simulink model "pendulum2d"  (R2017a)
settings: Solver=FixedStepAuto  StartTime=0.0  StopTime=10.0  FixedStep=1e-3  RelTol=1e-3
values from neighbouring files (symbols this model uses):
  theta_init = 15 *pi/180    (= 0.261799387799)    [initialize_2Dnonlinear_system.m]
libraries: sldrtlib x1
settings Model: Creator=Jan  LastModifiedBy=Jan

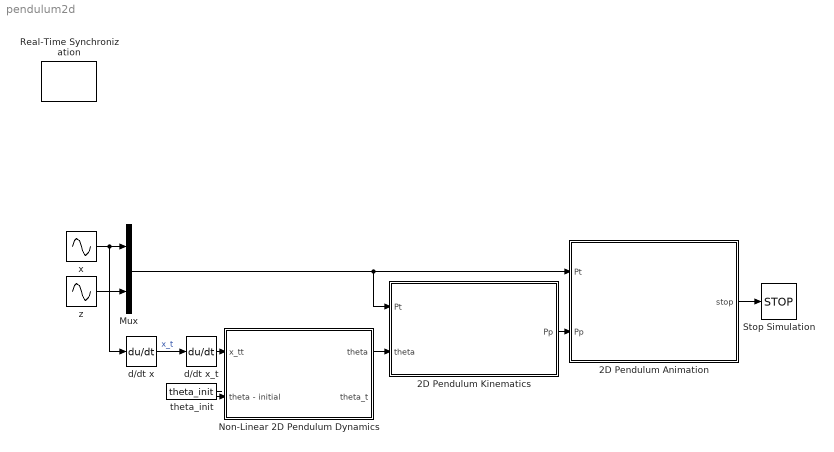
== system pendulum2d ==
  2D Pendulum Animation : MATLAB Function  TreatAsAtomicUnit=on  SystemSampleTime=0.05
  2D Pendulum Kinematics : MATLAB Function  TreatAsAtomicUnit=on
  Mux : Mux  Inputs=2
  Non-Linear 2D Pendulum Dynamics : Subsystem
  Real-Time Synchronization : sldrtlib/Real-Time Synchronization  SampleTime=0.05  MaxMissedTicks=10  ShowMissedTicks=off  YieldWhenWaiting=off
  Stop Simulation : Stop
  d/dt x : Derivative
  d/dt x_t : Derivative
  theta_init : Constant  Value=theta_init
  x : Sin  Frequency=2*pi*0.1  SampleTime=0
  z : Sin  Frequency=2*pi*0.1  SampleTime=0
  wires:
  theta_init/1 -> Non-Linear 2D Pendulum Dynamics/2(theta - initial)
  d/dt x_t/1 -> Non-Linear 2D Pendulum Dynamics/1(x_tt)
  d/dt x/1 -> d/dt x_t/1  "x_t"
  2D Pendulum Animation/1(stop) -> Stop Simulation/1
  x/1 -> d/dt x/1, Mux/1
  z/1 -> Mux/2
  Non-Linear 2D Pendulum Dynamics/1(theta) -> 2D Pendulum Kinematics/2(theta)
  Mux/1 -> 2D Pendulum Animation/1(Pt), 2D Pendulum Kinematics/1(Pt)
  2D Pendulum Kinematics/1(Pp) -> 2D Pendulum Animation/2(Pp)

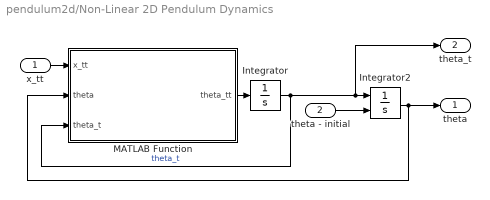
== system pendulum2d/Non-Linear 2D Pendulum Dynamics ==
  x_tt : Inport
  theta - initial : Inport  Port=2
  Integrator : Integrator
  Integrator2 : Integrator  InitialConditionSource=external
  MATLAB Function : MATLAB Function  TreatAsAtomicUnit=on
  theta : Outport
  theta_t : Outport  Port=2
  wires:
  Integrator2/1 -> theta/1, MATLAB Function/2(theta)
  theta - initial/1 -> Integrator2/2
  MATLAB Function/1(theta_tt) -> Integrator/1
  x_tt/1 -> MATLAB Function/1(x_tt)
  Integrator/1 -> theta_t/1, Integrator2/1, MATLAB Function/3(theta_t)  "theta_t"

== matlab function pendulum2d/Non-Linear 2D Pendulum Dynamics/MATLAB Function ==
  data: x_tt input; theta input; theta_tt output; theta_t input
function theta_tt = pendulum2D_dynamics(x_tt, theta, theta_t)
    
    % Constants
    g = 9.81;   % Gravity
    L = 2.0;    % Wire length
    
    % Pendulum ODE
    theta_tt = (-g*sin(theta) - cos(theta)*x_tt)/L;

== matlab function pendulum2d/2D Pendulum Kinematics ==
  data: Pt input; theta input; Pp output
function Pp = pendulum_kinematics(Pt, theta)
    
    % Constants
    g = 9.81;   % Gravity
    L = 2.0;    % Wire length
    
    % Pendulum Kinematics
    Pp = Pt + L*[sin(theta); -cos(theta)];

== matlab function pendulum2d/2D Pendulum Animation ==
  data: Pt input; stop output; Pp input
function stop = SimulinkPendulumPlot(Pt, Pp)
    % Creates a 2D-animation for the pendulum motion
    % Input:
    %   xt :   Position of tool-point
    %   theta : Euler angle of pendulum
    % Output:
    %   stop : Bool value to stop the animation
    
    % Persistent variables, to only be initialized once
    persistent h;           % Plot
    persistent L;
    
    stop = false;
    
    %% Initialization 
    % One time intitialization of plotting settings
    if isempty(h)
        % Plotting setup
        h = figure('Name','StewartPlatform Animation');
        L = 2.0;
        xlabel('x-axis')
        ylabel('y-axis')
%         zlabel('z-axis')
        xlim([-5, 5])
        ylim([-4, 1])
%         zlim([0, 8])
        hold on;
        grid on;
%         view(-40,20);
    end
    
     %% Drawing
    if ishandle(h)
        cla;
        plot_line(Pt, Pp);
        plot(Pp(1), Pp(2), 'ro', 'LineWidth', 2);

        drawnow;
    end
    
    %% Destructor
    if ~ishandle(h)
        stop = true;
    end

    function plot_line(p1, p2)
%         Pre-allocate
        line = zeros(2,2);
        line(1,:) = p1;
        line(2,:) = p2;

        plot(line(:,1), line(:,2), 'k')
    end
end
